simulink model "gm_soc_dvbs2_fpga"  (R2025b)
settings: Solver=VariableStepAuto  StartTime=0.0  StopTime=10.0  RelTol=1e-3
InitFcn:
  | soc_dvbs2_init;
undefined symbols (not defined in the file or in its folder): Add, coefficientsLog, coefficientsSqrt1, coefficientsSqrt2, dataBits, Deinterleaver, designMultirateFIR, noisePow, Shift, Short, soc_dvbs2_designFIRFilter, soc_dvbs2_txPacketBits, syncWord, txDataOut, txFiltCoeff, XData
libraries: simulink x304, hdlsllib x265, dspsigops x15, dsphdlfiltering2 x8, hdlmdlgenlib x6, dsphdlsigops2 x5, commseqgen3 x5, dsphdlmathfun2 x3, hwlogicconnlib x2, whdledac x2, commhdlcrc x2, whdlutilities x1
(part 2 of 36)

== system gm_soc_dvbs2_fpga/DVBS2/DVBS2 TxRx/LUT Based Tx ==
  modcodidx : Inport  OutDataTypeStr=fixdt(0, 5, 0)  PortDimensions=1  SampleTime=2.5e-07
  Constant : Constant  OutDataTypeStr=boolean  SampleTime=2.5e-07
  Data Type Conversion1 : DataTypeConversion  OutDataTypeStr=fixdt(1, 18, 15)  SampleTime=6.25e-08  SaturateOnIntegerOverflow=off  RndMeth=Floor
  Delay : Delay  DelayLength=double(2)  InitialCondition=0  SampleTime=2.5e-07
  Delay1 : Delay  DelayLength=double(1)  InitialCondition=0  SampleTime=2.5e-07
  Delay_out1_wire : RateTransition  Integrity=off  Deterministic=off  OutPortSampleTimeOpt=Multiple of input port sample time  OutPortSampleTimeMultiple=1/4
  Discrete FIR Filter HDL Optimized : dsphdlfiltering2/Discrete FIR Filter  NumeratorSource=Property  Numerator=txFiltCoeff  NumeratorPrototype=[]  FilterStructure=Direct form systolic  SerializationOption=Minimum number of cycles between valid input samples  NumCycles=2  NumberOfMultipliers=2  SimulateUsing=Code generation  roundingMode=Floor  overflowMode=off  CoefficientsDataTypeStr=Inherit: Same word length as input  OutputDataTypeStr=Inherit: Same word length as input  ResetInputPort=off  HDLGlobalReset=off  CoeffMultiplier=Multiplier  UseMultForPow2Coeff=on  FrameInputSymmOptim=off
  Subsystem1 : Subsystem
  Upsample : dspsigops/Upsample  FactorSource=Dialog parameter  N=double(4)  Nmax=16  phase=double(0)  RateOptions=Allow multirate processing  ic=0  mode=Unused parameter value
  txDataOut : Outport  SampleTime=6.25e-08
  txValidOut : Outport  Port=2  SampleTime=6.25e-08
  wires:
  Subsystem1/1(Out1) -> Delay1/1
  modcodidx/1 -> Subsystem1/1(modcodidx)
  Constant/1 -> Delay/1, Subsystem1/2(enb)
  Delay1/1 -> Upsample/1
  Delay_out1_wire/1 -> Discrete FIR Filter HDL Optimized/2
  Delay/1 -> Delay_out1_wire/1
  Discrete FIR Filter HDL Optimized/1 -> Data Type Conversion1/1
  Upsample/1 -> Discrete FIR Filter HDL Optimized/1
  Discrete FIR Filter HDL Optimized/2 -> txValidOut/1
  Data Type Conversion1/1 -> txDataOut/1

== system gm_soc_dvbs2_fpga/DVBS2/DVBS2 TxRx/Prepare Inputs ==
  rxData : Inport  OutDataTypeStr=int16  PortDimensions=1  SampleTime=7.8125e-09
      settings: SignalType=complex
  rxValid : Inport  Port=2  OutDataTypeStr=boolean  PortDimensions=1  SampleTime=7.8125e-09
  Data Type Conversion : DataTypeConversion  OutDataTypeStr=fixdt(1,16,14)  ConvertRealWorld=Stored Integer (SI)  SaturateOnIntegerOverflow=off  RndMeth=Floor
  Data Type Conversion1 : DataTypeConversion  OutDataTypeStr=fixdt(1,18,15)  ConvertRealWorld=Stored Integer (SI)  SaturateOnIntegerOverflow=off  RndMeth=Floor
  Delay{,1..3} (4 alike) : Delay
  Discrete FIR Filter HDL Optimized1 : dsphdlfiltering2/Discrete FIR Filter  NumeratorSource=Property  Numerator=soc_dvbs2_designFIRFilter(32,1.35,8-1.35)  NumeratorPrototype=[]  FilterStructure=Direct form systolic  SerializationOption=Minimum number of cycles between valid input samples  NumCycles=2  NumberOfMultipliers=2  SimulateUsing=Code generation  roundingMode=Floor  overflowMode=off  CoefficientsDataTypeStr=Inherit: Same word length as input  OutputDataTypeStr=Inherit: Same word length as input  ResetInputPort=off  HDLGlobalReset=off  CoeffMultiplier=Multiplier  UseMultForPow2Coeff=on  FrameInputSymmOptim=off
  Downsample1 : DownSample  N=8  RateOptions=Allow multirate processing
  Downsample2 : DownSample  N=8  RateOptions=Allow multirate processing
  Gain : Gain  Gain=2  ParamDataTypeStr=fixdt(0,3,0)  OutDataTypeStr=fixdt(1, 16, 13)
  rxDataOut : Outport  SampleTime=6.25e-08
  rxValidOut : Outport  Port=2  SampleTime=6.25e-08
  wires:
  rxData/1 -> Data Type Conversion/1
  Delay/1 -> Gain/1
  Downsample1/1 -> Delay1/1
  Delay2/1 -> Data Type Conversion1/1
  Discrete FIR Filter HDL Optimized1/1 -> Downsample2/1
  Gain/1 -> Delay2/1
  rxValid/1 -> Discrete FIR Filter HDL Optimized1/2
  Data Type Conversion/1 -> Discrete FIR Filter HDL Optimized1/1
  Downsample2/1 -> Delay/1
  Discrete FIR Filter HDL Optimized1/2 -> Downsample1/1
  Delay1/1 -> Delay3/1
  Delay3/1 -> rxValidOut/1
  Data Type Conversion1/1 -> rxDataOut/1

== system gm_soc_dvbs2_fpga/DVBS2/DVBS2 TxRx/Prepare Outputs ==
  note: Gain
  txData : Inport  OutDataTypeStr=fixdt(1, 18, 15)  PortDimensions=1  SampleTime=6.25e-08
      settings: SignalType=complex
  txvalid : Inport  Port=2  OutDataTypeStr=boolean  PortDimensions=1  SampleTime=6.25e-08
  Data Type Conversion2 : DataTypeConversion  OutDataTypeStr=int16  ConvertRealWorld=Stored Integer (SI)  SaturateOnIntegerOverflow=off  RndMeth=Floor
  Data Type Conversion3 : DataTypeConversion  OutDataTypeStr=fixdt(1,16,13)  SaturateOnIntegerOverflow=off  RndMeth=Floor
  Delay{4..7} (4 alike) : Delay
  Discrete FIR Filter HDL Optimized : dsphdlfiltering2/Discrete FIR Filter  NumeratorSource=Property  Numerator=soc_dvbs2_designFIRFilter(32,1.35,8-1.35)  NumeratorPrototype=[]  FilterStructure=Direct form systolic  SerializationOption=Minimum number of cycles between valid input samples  NumCycles=2  NumberOfMultipliers=2  SimulateUsing=Code generation  roundingMode=Floor  overflowMode=off  CoefficientsDataTypeStr=Inherit: Same word length as input  OutputDataTypeStr=Inherit: Same word length as input  ResetInputPort=off  HDLGlobalReset=off  CoeffMultiplier=Multiplier  UseMultForPow2Coeff=on  FrameInputSymmOptim=off
  Gain : Gain  Gain=8  ParamDataTypeStr=fixdt(0,4,0)  OutDataTypeStr=fixdt(1, 18, 14)
  Repeat : dspsigops/Repeat  FactorSource=Dialog parameter  N=8  Nmax=16  RateOptions=Allow multirate processing  ic=0  mode=Unused parameter value
  Upsample : dspsigops/Upsample  FactorSource=Dialog parameter  N=8  Nmax=16  phase=0  RateOptions=Allow multirate processing  ic=0  mode=Unused parameter value
  txDataOut : Outport  SampleTime=7.8125e-09
  txValidOut : Outport  Port=2  SampleTime=7.8125e-09
  wires:
  txData/1 -> Upsample/1
  txvalid/1 -> Repeat/1
  Delay6/1 -> Delay7/1
  Delay4/1 -> Gain/1
  Discrete FIR Filter HDL Optimized/2 -> Delay6/1
  Upsample/1 -> Discrete FIR Filter HDL Optimized/1
  Discrete FIR Filter HDL Optimized/1 -> Delay4/1
  Repeat/1 -> Discrete FIR Filter HDL Optimized/2
  Gain/1 -> Delay5/1
  Delay7/1 -> txValidOut/1
  Delay5/1 -> Data Type Conversion3/1
  Data Type Conversion3/1 -> Data Type Conversion2/1
  Data Type Conversion2/1 -> txDataOut/1

== system gm_soc_dvbs2_fpga/DVBS2/Vector Decimation/Vector Decimation ==
  din_real : Inport  OutDataTypeStr=int16  PortDimensions=[4]  SampleTime=7.8125e-09
  din_img : Inport  Port=2  OutDataTypeStr=int16  PortDimensions=[4]  SampleTime=7.8125e-09
  vin : Inport  Port=3  OutDataTypeStr=boolean  PortDimensions=1  SampleTime=7.8125e-09
  FIR Decimation HDL Optimized : dsphdlfiltering2/FIR Decimator  NumeratorSource=Property  Numerator=designMultirateFIR(1,4)  NumeratorPrototype=[]  FilterStructure=Direct form systolic  DecimationFactor=4  NumCycles=1  OptimizeSymmCoeff=off  SimulateUsing=Code generation  roundingMode=Floor  overflowMode=off  CoefficientsDataTypeStr=Inherit: Same word length as input  OutputDataTypeStr=fixdt(1,16,0)  ResetInputPort=off  HDLGlobalReset=off
  Real-Imag to Complex : RealImagToComplex
  dout : Outport  SampleTime=7.8125e-09  VectorParamsAs1DForOutWhenUnconnected=off
  vout : Outport  Port=2  SampleTime=7.8125e-09  VectorParamsAs1DForOutWhenUnconnected=off
  wires:
  FIR Decimation HDL Optimized/2 -> vout/1
  vin/1 -> FIR Decimation HDL Optimized/2
  din_real/1 -> Real-Imag to Complex/1
  FIR Decimation HDL Optimized/1 -> dout/1
  din_img/1 -> Real-Imag to Complex/2
  Real-Imag to Complex/1 -> FIR Decimation HDL Optimized/1

== system gm_soc_dvbs2_fpga/DVBS2/BER/Send Payload Data/1-D Lookup Table ==
  In1 : Inport
  1-D Lookup Table : Lookup_n-D  NumberOfTableDimensions=1  LookupTableObject=''  BreakpointsSpecification=Even spacing  BreakpointsForDimension1=0:length(dataBits)-1  BreakpointsForDimension1FirstPoint=0  BreakpointsForDimension2FirstPoint=10  BreakpointsForDimension2Spacing=12  IndexSearchMethod=Evenly spaced points  Table=[syncWord;soc_dvbs2_txPacketBits]  TableDataTypeStr=int8  InterpMethod=Flat  InternalRulePriority=Speed  OutDataTypeStr=int8  RndMeth=Simplest
  1-D Lookup Table_pd1 : Delay  DelayLength=1
  Out1 : Outport
  wires:
  1-D Lookup Table/1 -> 1-D Lookup Table_pd1/1
  In1/1 -> 1-D Lookup Table/1
  1-D Lookup Table_pd1/1 -> Out1/1

== system gm_soc_dvbs2_fpga/DVBS2/DVBS2 TxRx/Channel/AWGN Generator ==
  snrdB : Inport  OutDataTypeStr=fixdt(1, 16, 9)  PortDimensions=1  SampleTime=6.25e-08
  Delay1 : Delay  DelayLength=46
  Gaussian Noise With Given Variance : Subsystem
  Unit Variance Gaussian Noise : Subsystem
  dB to Linear Scale Converter : Subsystem
  awgn : Outport  SampleTime=6.25e-08
  wires:
  snrdB/1 -> dB to Linear Scale Converter/1(snrdB)
  dB to Linear Scale Converter/1(noiseVar) -> Delay1/1
  Gaussian Noise With Given Variance/1(awgn) -> awgn/1
  Unit Variance Gaussian Noise/1(x0) -> Gaussian Noise With Given Variance/2(x0)
  Delay1/1 -> Gaussian Noise With Given Variance/1(noiseVar)
  Unit Variance Gaussian Noise/2(x1) -> Gaussian Noise With Given Variance/3(x1)

== system gm_soc_dvbs2_fpga/DVBS2/DVBS2 TxRx/DVB-S2 HDL Receiver/Demod Deinterleave and FECDecode ==
  dataIn : Inport  OutDataTypeStr=fixdt(1, 18, 14)  PortDimensions=1  SampleTime=7.8125e-09
      settings: SignalType=complex
  validIn : Inport  Port=2  OutDataTypeStr=boolean  PortDimensions=1  SampleTime=7.8125e-09
  endOfPLSC : Inport  Port=3  OutDataTypeStr=boolean  PortDimensions=1  SampleTime=7.8125e-09
  MODCOD : Inport  Port=4  OutDataTypeStr=fixdt(0, 5, 0)  PortDimensions=1  SampleTime=7.8125e-09
  DVBS2 HDL Deinterleaver : Subsystem  mask{mode=Deinterleaver, Tsamp=double(-1)}
      mask prompts: mode "Mode :"; Tsamp "Sample Time"
      mask init:
      | ConfigRx = struct('RAMCapacity', double(129600), 'ShortFrameLen', double(16200), 'NormalFrameLen', double(64800));
      | Tsamp = double(-1);
      | isInterleave = double(0);
      mask TypeOptions mode: Interleaver | Deinterleaver
      mask Display: disp(['DVB-S2' newline 'HDL ' newline get_param(gcb,'mode')]);
  Data Type Conversion3 : DataTypeConversion  OutDataTypeStr=fixdt(1,8,4)  RndMeth=Floor
  Discard Unsupported Frames : Subsystem
  FEC Decoding : Subsystem
  Symbol Demodulaor : Subsystem
  bitsOut : Outport  SampleTime=7.8125e-09
  ctrl : Outport  Port=2
  wires:
  MODCOD/1 -> Discard Unsupported Frames/4(MODCOD)
  validIn/1 -> Discard Unsupported Frames/3(validIn)
  dataIn/1 -> Discard Unsupported Frames/2(dataIn)
  endOfPLSC/1 -> Discard Unsupported Frames/1(endOfPLSC)
  Data Type Conversion3/1 -> DVBS2 HDL Deinterleaver/1(dataIn)
  Discard Unsupported Frames/4(modIdx) -> Symbol Demodulaor/4(modIdx)
  Discard Unsupported Frames/3(paramCapture) -> Symbol Demodulaor/3(paramCapture)
  Discard Unsupported Frames/2(validOut) -> Symbol Demodulaor/2(validIn)
  Discard Unsupported Frames/1(dataOut) -> Symbol Demodulaor/1(dataIn)
  Discard Unsupported Frames/5(codIdx) -> Symbol Demodulaor/5(codIdx)
  Discard Unsupported Frames/6(FECFrameOut) -> Symbol Demodulaor/6(FECFrame)
  Symbol Demodulaor/1(softBitsOut) -> Data Type Conversion3/1
  Symbol Demodulaor/2(validOut) -> DVBS2 HDL Deinterleaver/2(validIn)
  Symbol Demodulaor/3(paramCaptureOut) -> DVBS2 HDL Deinterleaver/3(paramValid)
  Symbol Demodulaor/4(modIdxOut) -> DVBS2 HDL Deinterleaver/4(modIdxIn)
  Symbol Demodulaor/5(codIdxOut) -> DVBS2 HDL Deinterleaver/5(codIdxIn)
  Symbol Demodulaor/6(fecframeOut) -> DVBS2 HDL Deinterleaver/6(fecframeIn)
  DVBS2 HDL Deinterleaver/1(rd_dout) -> FEC Decoding/1(dataIn)
  DVBS2 HDL Deinterleaver/2(rd_startOut) -> FEC Decoding/2(startIn)
  DVBS2 HDL Deinterleaver/3(rd_endOut) -> FEC Decoding/3(endIn)
  DVBS2 HDL Deinterleaver/4(rd_validOut) -> FEC Decoding/4(validIn)
  DVBS2 HDL Deinterleaver/5(fecframe) -> FEC Decoding/5(FECFrame)
  FEC Decoding/2(ctrl) -> ctrl/1
  DVBS2 HDL Deinterleaver/6(codIdx) -> FEC Decoding/6(codIdx)
  FEC Decoding/1(bitsOut) -> bitsOut/1

== system gm_soc_dvbs2_fpga/DVBS2/DVBS2 TxRx/DVB-S2 HDL Receiver/Stream Recovery ==
  bitsIn : Inport  OutDataTypeStr=boolean  PortDimensions=1  SampleTime=7.8125e-09
  startIn : Inport  Port=2  OutDataTypeStr=boolean  PortDimensions=1  SampleTime=7.8125e-09
  validIn : Inport  Port=3  OutDataTypeStr=boolean  PortDimensions=1  SampleTime=7.8125e-09
  BB Decoder : Subsystem
  BB Demultiplexer : Subsystem
  BB Descrambler : Subsystem
  BB Header CRC Check : Subsystem
  Delay{1..2,4..9,11..15,17..18,20..24} (20 alike) : Delay  DelayLength=1
  bitsOut : Outport  OutDataTypeStr=boolean  PortDimensions=[1 1]  SampleTime=7.8125e-09
  startOut : Outport  Port=2  OutDataTypeStr=boolean  PortDimensions=[1 1]  SampleTime=7.8125e-09
  endOut : Outport  Port=3  OutDataTypeStr=boolean  PortDimensions=[1 1]  SampleTime=7.8125e-09
  validOut : Outport  Port=4  OutDataTypeStr=boolean  PortDimensions=[1 1]  SampleTime=7.8125e-09
  invalidPkt : Outport  Port=5  OutDataTypeStr=boolean  PortDimensions=[1 1]  SampleTime=7.8125e-09
  TSorGS : Outport  Port=6  OutDataTypeStr=fixdt(0,2,0)  PortDimensions=[1 1]  SampleTime=7.8125e-09
  SISorMIS : Outport  Port=7  OutDataTypeStr=boolean  PortDimensions=[1 1]  SampleTime=7.8125e-09
  CCMorACM : Outport  Port=8  OutDataTypeStr=boolean  PortDimensions=[1 1]  SampleTime=7.8125e-09
  ISSYI : Outport  Port=9  OutDataTypeStr=boolean  PortDimensions=[1 1]  SampleTime=7.8125e-09
  NPD : Outport  Port=10  OutDataTypeStr=boolean  PortDimensions=[1 1]  SampleTime=7.8125e-09
  RO : Outport  Port=11  OutDataTypeStr=fixdt(0,2,0)  PortDimensions=[1 1]  SampleTime=7.8125e-09
  MIS_ISI : Outport  Port=12  OutDataTypeStr=uint8  PortDimensions=1  SampleTime=7.8125e-09
  UPL : Outport  Port=13  OutDataTypeStr=uint16  PortDimensions=1  SampleTime=7.8125e-09
  DFL : Outport  Port=14  OutDataTypeStr=uint16  PortDimensions=1  SampleTime=7.8125e-09
  SYNC : Outport  Port=15  OutDataTypeStr=uint8  PortDimensions=1  SampleTime=7.8125e-09
  SYNCD : Outport  Port=16  OutDataTypeStr=uint16  PortDimensions=1  SampleTime=7.8125e-09
  wires:
  Delay6/1 -> BB Descrambler/3(validIn)
  BB Header CRC Check/1(dstartOut) -> Delay9/1
  bitsIn/1 -> Delay1/1
  startIn/1 -> Delay2/1
  validIn/1 -> Delay6/1
  Delay17/1 -> BB Demultiplexer/3(validIn)
  BB Descrambler/1(bitsOut) -> Delay7/1
  Delay1/1 -> BB Descrambler/1(bitsIn)
  Delay2/1 -> BB Descrambler/2(startIn)
  Delay15/1 -> BB Demultiplexer/2(startIn)
  BB Descrambler/2(startOut) -> Delay15/1
  BB Descrambler/3(validOut) -> Delay17/1
  Delay7/1 -> BB Demultiplexer/1(bitsIn)
  BB Decoder/5(TSorGS) -> TSorGS/1
  BB Demultiplexer/1(dstartOut) -> Delay18/1
  BB Decoder/12(UPL) -> UPL/1
  BB Demultiplexer/2(dValidOut) -> Delay20/1
  BB Decoder/15(SYNCD) -> SYNCD/1
  BB Demultiplexer/3(bitsOut) -> Delay21/1
  BB Decoder/6(SISorMIS) -> SISorMIS/1
  BB Demultiplexer/4(hstartOut) -> Delay22/1
  BB Decoder/9(NPD) -> NPD/1
  BB Demultiplexer/5(hendOut) -> Delay23/1
  BB Decoder/8(ISSYI) -> ISSYI/1
  BB Demultiplexer/6(hvalidOut) -> Delay24/1
  Delay18/1 -> BB Header CRC Check/1(dstartIn)
  Delay11/1 -> BB Decoder/2(dvalidIn)
  Delay20/1 -> BB Header CRC Check/2(dValidIn)
  Delay21/1 -> BB Header CRC Check/3(bitsIn)
  Delay9/1 -> BB Decoder/1(dstartIn)
  Delay22/1 -> BB Header CRC Check/4(hstartIn)
  Delay23/1 -> BB Header CRC Check/5(hendIn)
  Delay24/1 -> BB Header CRC Check/6(hvalidIn)
  BB Header CRC Check/2(dvalidIn) -> Delay11/1
  BB Header CRC Check/3(dbitsOut) -> Delay8/1
  BB Header CRC Check/4(hbitsOut) -> Delay13/1
  BB Header CRC Check/5(hstartOut) -> Delay4/1
  BB Header CRC Check/6(hendOut) -> Delay5/1
  BB Header CRC Check/7(hvalidOut) -> Delay12/1
  Delay5/1 -> BB Decoder/6(hendIn)
  BB Header CRC Check/8(herrorOut) -> Delay14/1
  Delay8/1 -> BB Decoder/3(dbitsIn)
  Delay13/1 -> BB Decoder/4(hbitsIn)
  Delay4/1 -> BB Decoder/5(hstartIn)
  Delay12/1 -> BB Decoder/7(validIn)
  Delay14/1 -> BB Decoder/8(herrorIn)
  BB Decoder/1(bitsOut) -> bitsOut/1
  BB Decoder/2(startOut) -> startOut/1
  BB Decoder/3(endOut) -> endOut/1
  BB Decoder/4(validOut) -> validOut/1
  BB Decoder/7(CCMorACM) -> CCMorACM/1
  BB Decoder/10(RO) -> RO/1
  BB Decoder/11(MIS_ISI) -> MIS_ISI/1
  BB Decoder/13(DFL) -> DFL/1
  BB Decoder/14(SYNC) -> SYNC/1
  BB Decoder/16(invalidPkt) -> invalidPkt/1

== system gm_soc_dvbs2_fpga/DVBS2/DVBS2 TxRx/DVB-S2 HDL Receiver/Synchronizer and PL Header Decoder ==
  dataIn : Inport  OutDataTypeStr=fixdt(1, 18, 15)  PortDimensions=1  SampleTime=6.25e-08
      settings: SignalType=complex
  validIn : Inport  Port=2  OutDataTypeStr=boolean  PortDimensions=1  SampleTime=6.25e-08
  rstFCPO : Inport  Port=3  OutDataTypeStr=boolean  PortDimensions=1  SampleTime=6.25e-08
  Bus Creator : BusCreator  Inputs=2
  Bus Creator1 : BusCreator  Inputs=2
  Bus Creator2 : BusCreator  Inputs=5
  Delay10 : Delay  DelayLength=6
  Delay{3,11,13..21,24} (12 alike) : Delay  DelayLength=1
  Delay{4..7,12} (5 alike) : Delay
  Delay9 : Delay  DelayLength=6
  Downsample : DownSample  N=config.SamplesPerSymbol  RateOptions=Allow multirate processing
  "Enable MODCOD " : Subsystem
  Fine Phase Synchronizer : Subsystem
  PL Header Recovery : Subsystem
  Source Encoding : Subsystem
  Time Frequency and Coarse Phase Synchronizer : Subsystem
  dataOut : Outport  SampleTime=2.5e-07
  validOut : Outport  Port=2  SampleTime=2.5e-07
  endOfPLSC : Outport  Port=3  SampleTime=2.5e-07
  headerInfo : Outport  Port=4
  diagBus : Outport  Port=5
  wires:
  [diagBus3] -> Bus Creator2/3  "SymbolSyncedSymbols"
  dataIn/1 -> Delay20/1
  Delay7/1 -> Delay10/1
  [diagBus1] -> Bus Creator2/1  "PLSCSymbols"
  [diagBus5] -> Bus Creator2/5  "VisualizeCorrelationSignals"
  Downsample/1 -> Fine Phase Synchronizer/6(rst)
  [diagBus4] -> Bus Creator2/4  "pilotsConstellation"
  [diagBus2] -> Bus Creator2/2  "NormalizedFrequencyEstimates"
  Bus Creator2/1 -> Delay11/1
  PL Header Recovery/4(endOfPLSC) -> Delay5/1
  Time Frequency and Coarse Phase Synchronizer/3(validOut) -> Delay14/1
  validIn/1 -> Delay3/1
  Delay20/1 -> Time Frequency and Coarse Phase Synchronizer/1(dataIn)
  Delay3/1 -> Time Frequency and Coarse Phase Synchronizer/2(validIn)
  Source Encoding/1(mod) -> Fine Phase Synchronizer/4(mod)
  Delay15/1 -> PL Header Recovery/3(endOfSOF)
  Delay11/1 -> diagBus/1
  Delay4/1 -> Fine Phase Synchronizer/2(validIn)
  PL Header Recovery/2(dataOut) -> Delay12/1
  Time Frequency and Coarse Phase Synchronizer/1(finePhaseEn) -> Fine Phase Synchronizer/5(En)
  Time Frequency and Coarse Phase Synchronizer/2(dataOut) -> Delay13/1
  Time Frequency and Coarse Phase Synchronizer/4(endOfSOF) -> Delay15/1
  Time Frequency and Coarse Phase Synchronizer/5(hasPilots) -> Delay16/1
  Time Frequency and Coarse Phase Synchronizer/6(normCoarFreqEst) -> Bus Creator/1  "NormalizedCoarseFrequencyEstimate"
  Time Frequency and Coarse Phase Synchronizer/7(normFineFreqEst) -> Bus Creator/2  "NormalizedFineFrequencyEstimate"
  Time Frequency and Coarse Phase Synchronizer/8(synbSyncDiag) -> [diagBus3]
  Time Frequency and Coarse Phase Synchronizer/9(pilotConstel) -> [diagBus4]
  Time Frequency and Coarse Phase Synchronizer/10(VisualizeCorrelationSignals) -> [diagBus5]
  Time Frequency and Coarse Phase Synchronizer/11(enbMODCOD) -> "Enable MODCOD "/2(enb)
  Delay13/1 -> PL Header Recovery/1(dataIn)
  Delay14/1 -> PL Header Recovery/2(validIn)
  Delay16/1 -> PL Header Recovery/4(hasPilots)
  PL Header Recovery/5(modcod) -> Source Encoding/1(modcod), Delay6/1
  Bus Creator/1 -> [diagBus2]
  Bus Creator1/1 -> Delay21/1
  Delay5/1 -> Fine Phase Synchronizer/3(endOfPLSCIn)
  PL Header Recovery/1(PLSCDiag) -> [diagBus1]
  rstFCPO/1 -> Delay24/1
  PL Header Recovery/3(validOut) -> Delay4/1
  Delay9/1 -> "Enable MODCOD "/1(modcod)
  PL Header Recovery/6(FEC) -> Delay7/1
  Delay24/1 -> Downsample/1
  Delay12/1 -> Fine Phase Synchronizer/1(dataIn)
  Delay6/1 -> Delay9/1
  Fine Phase Synchronizer/1(dataOut) -> Delay17/1
  Fine Phase Synchronizer/2(validOut) -> Delay18/1
  Fine Phase Synchronizer/3(endOfPLSC) -> Delay19/1
  Delay10/1 -> Bus Creator1/2  "FECFrame"
  Delay17/1 -> dataOut/1
  Delay18/1 -> validOut/1
  Delay19/1 -> endOfPLSC/1
  "Enable MODCOD "/1(modcodOut) -> Bus Creator1/1  "MODCOD"
  Delay21/1 -> headerInfo/1

== system gm_soc_dvbs2_fpga/DVBS2/DVBS2 TxRx/Digital Automatic Gain Control/Error Detector ==
  dataIn : Inport  OutDataTypeStr=fixdt(1, 18, 15)  PortDimensions=1  SampleTime=6.25e-08
      settings: SignalType=complex
  Add1 : Sum  Inputs=+-  OutDataTypeStr=fixdt(1, 37, 30)
  Complex to Real-Imag : ComplexToRealImag  Output=Real
  Conj : Math  Operator=conj  OutDataTypeStr=fixdt(1, 18, 15)
  Delay{,1,3..4} (4 alike) : Delay
  Product : Product  OutDataTypeStr=fixdt(1, 36, 30)
  Reference : Constant  Value=desiredOutputPower  OutDataTypeStr=fixdt(1, 18, 15)  SampleTime=-1
  err : Outport  SampleTime=6.25e-08
  wires:
  dataIn/1 -> Delay1/1, Conj/1
  Reference/1 -> Add1/1
  Conj/1 -> Delay/1
  Delay4/1 -> Complex to Real-Imag/1
  Product/1 -> Delay4/1
  Add1/1 -> Delay3/1
  Delay1/1 -> Product/1
  Delay3/1 -> err/1
  Complex to Real-Imag/1 -> Add1/2
  Delay/1 -> Product/2

== system gm_soc_dvbs2_fpga/DVBS2/DVBS2 TxRx/Digital Automatic Gain Control/Loop Filter ==
  err : Inport  OutDataTypeStr=fixdt(1, 37, 30)  PortDimensions=1  SampleTime=6.25e-08
  Add : Sum  OutDataTypeStr=fixdt(1, 37, 30)  AccumDataTypeStr=fixdt(1, 38, 30)  SampleTime=6.25e-08
  Delay1 : Delay  DelayLength=double(1)  InitialCondition=0  SampleTime=6.25e-08
  Delay2 : Delay  DelayLength=double(2)  InitialCondition=0  SampleTime=6.25e-08
  Delay3 : Delay  DelayLength=double(2)  InitialCondition=0  SampleTime=6.25e-08
  Gain1 : Gain  Gain="fi(0,1,37,46,\"hex\",\"083126e979\")"  ParamDataTypeStr=fixdt(1, 37, 46)  OutDataTypeStr=fixdt(1, 37, 30)  SampleTime=6.25e-08
  gain : Outport  SampleTime=6.25e-08
  wires:
  err/1 -> Delay3/1
  Delay1/1 -> gain/1, Add/2
  Delay3/1 -> Gain1/1
  Add/1 -> Delay1/1
  Gain1/1 -> Delay2/1
  Delay2/1 -> Add/1

== system gm_soc_dvbs2_fpga/DVBS2/DVBS2 TxRx/LUT Based Tx/Subsystem1 ==
  modcodidx : Inport  OutDataTypeStr=fixdt(0, 5, 0)  PortDimensions=1  SampleTime=2.5e-07
  enb : Inport  Port=2  OutDataTypeStr=boolean  PortDimensions=1  SampleTime=2.5e-07
  Delay : Delay  DelayLength=double(1)  InitialCondition=0  SampleTime=2.5e-07
  From : hdlmdlgenlib/Buffer
  Goto : hdlmdlgenlib/Buffer
  Logical Operator : Logic  Operator=OR  Inputs=4  AllPortsSameDT=off  OutDataTypeStr=boolean  SampleTime=2.5e-07
  Multiport Switch : MultiPortSwitch  DataPortOrder=Zero-based contiguous  Inputs=24  DataPortForDefault=Additional data port  DiagnosticForDefault=None  zeroidx=on  OutDataTypeStr=fixdt(1, 18, 16)  SampleTime=2.5e-07  SaturateOnIntegerOverflow=off  InputSameDT=off
  Subsystem : Subsystem
  Subsystem1 : Subsystem
  Subsystem2 : Subsystem
  Subsystem4 : Subsystem
  Unit Delay Enabled Synchronous : hdlsllib/Discrete/Unit Delay Enabled Synchronous  InitialCondition=double(0)  SampleTime=-1
  delayMatch : Delay  DelayLength=double(1)  InitialCondition=0  SampleTime=2.5e-07
  Out1 : Outport  SampleTime=2.5e-07
  wires:
  Subsystem/2(Out3) -> Multiport Switch/3
  Subsystem/6(Out7) -> Multiport Switch/7
  modcodidx/1 -> Unit Delay Enabled Synchronous/1
  From/1 -> Subsystem1/3(modcodidx), Subsystem/3(modcodidx), Subsystem4/3(modcodidx), Subsystem2/3(modcodidx)
  Subsystem4/7(Out1) -> Logical Operator/2
  Goto/1 -> From/1
  Unit Delay Enabled Synchronous/1 -> delayMatch/1, Goto/1
  delayMatch/1 -> Multiport Switch/1
  Subsystem/1(Out2) -> Multiport Switch/26, Multiport Switch/2
  Subsystem/5(Out6) -> Multiport Switch/6
  enb/1 -> Subsystem2/2(enb), Subsystem4/2(enb), Subsystem1/2(enb), Subsystem/2(enb)
  Subsystem/3(Out4) -> Multiport Switch/4
  Subsystem/4(Out5) -> Multiport Switch/5
  Subsystem/7(Out1) -> Logical Operator/1
  Subsystem1/1(Out2) -> Multiport Switch/8
  Subsystem1/2(Out3) -> Multiport Switch/9
  Subsystem1/3(Out4) -> Multiport Switch/10
  Subsystem1/4(Out5) -> Multiport Switch/11
  Subsystem1/5(Out6) -> Multiport Switch/12
  Subsystem1/6(Out7) -> Multiport Switch/13
  Subsystem1/7(Out1) -> Logical Operator/3
  Subsystem4/1(Out2) -> Multiport Switch/14
  Subsystem4/2(Out3) -> Multiport Switch/15
  Subsystem4/3(Out4) -> Multiport Switch/16
  Subsystem4/4(Out5) -> Multiport Switch/17
  Subsystem4/5(Out6) -> Multiport Switch/18
  Subsystem4/6(Out7) -> Multiport Switch/19
  Subsystem2/1(Out2) -> Multiport Switch/20
  Delay/1 -> Subsystem2/1(rst), Subsystem4/1(rst), Subsystem/1(rst), Subsystem1/1(rst)
  Subsystem2/2(Out3) -> Multiport Switch/21
  Subsystem2/3(Out4) -> Multiport Switch/22
  Subsystem2/4(Out5) -> Multiport Switch/23
  Subsystem2/5(Out6) -> Multiport Switch/24
  Subsystem2/6(Out7) -> Multiport Switch/25
  Subsystem2/7(Out1) -> Logical Operator/4
  Multiport Switch/1 -> Out1/1
  Logical Operator/1 -> Unit Delay Enabled Synchronous/2, Delay/1

== system gm_soc_dvbs2_fpga/DVBS2/DVBS2 TxRx/Channel/AWGN Generator/Gaussian Noise With Given Variance ==
  noiseVar : Inport  OutDataTypeStr=fixdt(0, 22, 18)  PortDimensions=1  SampleTime=6.25e-08
  x0 : Inport  Port=2  OutDataTypeStr=fixdt(1, 16, 11)  PortDimensions=1  SampleTime=6.25e-08
  x1 : Inport  Port=3  OutDataTypeStr=fixdt(1, 16, 11)  PortDimensions=1  SampleTime=6.25e-08
  Add1 : Sum  OutDataTypeStr=fixdt(1, 16, 11)  AccumDataTypeStr=fixdt(1, 33, 25)  SampleTime=6.25e-08
  Delay{1..9} (9 alike) : Delay  DelayLength=double(2)  InitialCondition=0  SampleTime=6.25e-08
  Gain : Gain  Gain="fi(0,1,16,14,\"hex\",\"0000 + 4000 i\")"  ParamDataTypeStr=fixdt(1, 16, 14)  OutDataTypeStr=fixdt(1, 32, 25)  SampleTime=6.25e-08
  Product1 : Product  Inputs=**  OutDataTypeStr=fixdt(1, 38, 29)  SampleTime=6.25e-08
  Product11 : Product  Inputs=**  OutDataTypeStr=fixdt(1, 38, 29)  SampleTime=6.25e-08
  Product1_C2ReIm : ComplexToRealImag  SampleTime=6.25e-08
  Product1_ReIm2Complex : RealImagToComplex  SampleTime=6.25e-08
  awgn : Outport  SampleTime=6.25e-08
  wires:
  Delay5/1 -> Add1/2
  x1/1 -> Delay9/1
  Delay4/1 -> Add1/1
  Delay3/1 -> Product1_C2ReIm/1
  x0/1 -> Delay8/1
  Product11/1 -> Product1_ReIm2Complex/2
  Product1_C2ReIm/2 -> Product11/1
  Gain/1 -> Delay5/1
  Delay8/1 -> Delay4/1
  Delay9/1 -> Gain/1
  noiseVar/1 -> Delay7/1
  Product1_ReIm2Complex/1 -> Delay1/1
  Product1/1 -> Product1_ReIm2Complex/1
  Add1/1 -> Delay3/1
  Delay7/1 -> Delay6/1
  Delay6/1 -> Delay2/1
  Product1_C2ReIm/1 -> Product1/1
  Delay2/1 -> Product11/2, Product1/2
  Delay1/1 -> awgn/1

== system gm_soc_dvbs2_fpga/DVBS2/DVBS2 TxRx/Channel/AWGN Generator/Unit Variance Gaussian Noise ==
  Delay{,1..2,31,33} (5 alike) : Delay  DelayLength=double(1)  InitialCondition=0  SampleTime=6.25e-08
  Delay{5..10} (6 alike) : Delay  DelayLength=double(2)  InitialCondition=0  SampleTime=6.25e-08
  Delay23 : Delay  DelayLength=double(19)  InitialCondition=0  SampleTime=6.25e-08
  Delay24 : Delay  DelayLength=double(19)  InitialCondition=0  SampleTime=6.25e-08
  Delay3 : Delay  DelayLength=double(21)  InitialCondition=0  SampleTime=6.25e-08
  Delay4 : Delay  DelayLength=double(21)  InitialCondition=0  SampleTime=6.25e-08
  Product : Product  Inputs=**  OutDataTypeStr=fixdt(1, 33, 28)  SampleTime=6.25e-08
  Product1 : Product  Inputs=**  OutDataTypeStr=fixdt(1, 33, 28)  SampleTime=6.25e-08
  Product1_out_dtc : DataTypeConversion  OutDataTypeStr=fixdt(1, 16, 11)  SampleTime=6.25e-08  SaturateOnIntegerOverflow=off  RndMeth=Floor
  Product_out_dtc : DataTypeConversion  OutDataTypeStr=fixdt(1, 16, 11)  SampleTime=6.25e-08  SaturateOnIntegerOverflow=off  RndMeth=Floor
  SinCos : Subsystem
  SqrtImplementation : Subsystem
  TausUniformRandGen : Subsystem
  logImplementation : Subsystem
  x0 : Outport  SampleTime=6.25e-08
  x1 : Outport  Port=2  SampleTime=6.25e-08
  wires:
  TausUniformRandGen/1(u0(16,16)) -> Delay/1
  Delay1/1 -> SqrtImplementation/1(u)
  Delay/1 -> logImplementation/1(u0(48,48))
  TausUniformRandGen/2(u1(16,16)) -> Delay2/1
  Delay2/1 -> SinCos/1(u1)
  logImplementation/1(e) -> Delay1/1
  SinCos/2(g1(16,15)) -> Delay4/1
  SinCos/1(g0) -> Delay3/1
  Delay9/1 -> x0/1
  SqrtImplementation/1(f) -> Delay7/1, Delay5/1
  Delay3/1 -> Delay31/1
  Delay4/1 -> Delay33/1
  Delay31/1 -> Delay23/1
  Delay33/1 -> Delay24/1
  Delay23/1 -> Delay6/1
  Delay8/1 -> Product1/2
  Delay24/1 -> Delay8/1
  Delay5/1 -> Product/1
  Delay6/1 -> Product/2
  Delay7/1 -> Product1/1
  Product/1 -> Product_out_dtc/1
  Product1/1 -> Product1_out_dtc/1
  Product_out_dtc/1 -> Delay9/1
  Product1_out_dtc/1 -> Delay10/1
  Delay10/1 -> x1/1

== system gm_soc_dvbs2_fpga/DVBS2/DVBS2 TxRx/Channel/AWGN Generator/dB to Linear Scale Converter ==
  snrdB : Inport  OutDataTypeStr=fixdt(1, 16, 9)  PortDimensions=1  SampleTime=6.25e-08
  Add : Sum  OutDataTypeStr=int16  AccumDataTypeStr=int16  SampleTime=6.25e-08
  Constant : Constant  Value=201  OutDataTypeStr=int16  SampleTime=6.25e-08
  Delay{1..4} (4 alike) : Delay  DelayLength=double(2)  InitialCondition=0  SampleTime=6.25e-08
  Delay5 : Delay  DelayLength=double(1)  InitialCondition=0  SampleTime=6.25e-08
  Delay6 : Delay  DelayLength=double(1)  InitialCondition=0  SampleTime=6.25e-08
  Gain : Gain  Gain="fi(0,1,16,11,\"hex\",\"5000\")"  ParamDataTypeStr=fixdt(1, 16, 11)  OutDataTypeStr=fixdt(1, 32, 20)  SampleTime=6.25e-08
  Gain_out_dtc : DataTypeConversion  OutDataTypeStr=int16  RndMeth=Round  SampleTime=6.25e-08  SaturateOnIntegerOverflow=off
  sqrt(noisePow/2) : Lookup_n-D  NumberOfTableDimensions=1  LookupTableObject=''  BreakpointsForDimension1=0:511  BreakpointsForDimension1FirstPoint=10  BreakpointsForDimension2FirstPoint=10  BreakpointsForDimension1Spacing=12  BreakpointsForDimension2Spacing=12  IndexSearchMethod=Evenly spaced points  Table=[0 noisePow]  InterpMethod=Flat  InternalRulePriority=Speed  OutDataTypeStr=fixdt(0,22,18)  RndMeth=Simplest
  noiseVar : Outport  SampleTime=6.25e-08
  wires:
  Constant/1 -> Add/2
  Delay3/1 -> Add/1
  Delay2/1 -> Gain/1
  snrdB/1 -> Delay5/1
  Add/1 -> Delay1/1
  Gain_out_dtc/1 -> Delay3/1
  Gain/1 -> Gain_out_dtc/1
  Delay5/1 -> Delay2/1
  Delay1/1 -> sqrt(noisePow/2)/1
  sqrt(noisePow/2)/1 -> Delay4/1
  Delay4/1 -> Delay6/1
  Delay6/1 -> noiseVar/1

== system gm_soc_dvbs2_fpga/DVBS2/DVBS2 TxRx/DVB-S2 HDL Receiver/Demod Deinterleave and FECDecode/DVBS2 HDL Deinterleaver ==
  dataIn : Inport  OutDataTypeStr=fixdt(1, 8, 4)  PortDimensions=1  SampleTime=7.8125e-09
  validIn : Inport  Port=2  OutDataTypeStr=boolean  PortDimensions=1  SampleTime=7.8125e-09
  paramValid : Inport  Port=3  OutDataTypeStr=boolean  PortDimensions=1  SampleTime=7.8125e-09
  modIdxIn : Inport  Port=4  OutDataTypeStr=fixdt(0, 2, 0)  PortDimensions=1  SampleTime=7.8125e-09
  codIdxIn : Inport  Port=5  OutDataTypeStr=fixdt(0, 4, 0)  PortDimensions=1  SampleTime=7.8125e-09
  fecframeIn : Inport  Port=6  OutDataTypeStr=boolean  PortDimensions=1  SampleTime=7.8125e-09
  Constant1 : Constant  Value=0  OutDataTypeStr=fixdt(1, 8, 4)  SampleTime=Tsamp
  Delay{,1..15,20..23} (20 alike) : Delay  DelayLength=1
  Delay16 : Delay  DelayLength=4
  Delay17 : Delay  DelayLength=4
  Discard Out of  Frame samples : Subsystem
  RAM : Subsystem
  RAM Address Generator : Subsystem
  Switch : Switch  Criteria=u2 > Threshold  OutDataTypeStr=fixdt(1, 8, 4)  SaturateOnIntegerOverflow=off  InputSameDT=off
  Unit Delay Enabled Synchronous : hdlsllib/Discrete/Unit Delay Enabled Synchronous  InitialCondition=0.0  SampleTime=-1
  Unit Delay Enabled Synchronous1 : hdlsllib/Discrete/Unit Delay Enabled Synchronous  InitialCondition=0.0  SampleTime=-1
  Unit Delay Enabled Synchronous2 : hdlsllib/Discrete/Unit Delay Enabled Synchronous  InitialCondition=0.0  SampleTime=-1
  codIdxReg : hdlsllib/Discrete/Unit Delay Enabled Synchronous  InitialCondition=0.0  SampleTime=-1
  fecframeReg : hdlsllib/Discrete/Unit Delay Enabled Synchronous  InitialCondition=0.0  SampleTime=-1
  rd_dout : Outport  SampleTime=7.8125e-09
  rd_startOut : Outport  Port=2  SampleTime=7.8125e-09
  rd_endOut : Outport  Port=3  SampleTime=7.8125e-09
  rd_validOut : Outport  Port=4  SampleTime=7.8125e-09
  fecframe : Outport  Port=5  SampleTime=7.8125e-09
  codIdx : Outport  Port=6  SampleTime=7.8125e-09
  wires:
  codIdxIn/1 -> Unit Delay Enabled Synchronous2/1
  Delay15/1 -> fecframeReg/1
  fecframeIn/1 -> Unit Delay Enabled Synchronous1/1
  validIn/1 -> Discard Out of  Frame samples/2(valid)
  Delay10/1 -> RAM/4(rd_addr)
  dataIn/1 -> Discard Out of  Frame samples/1(dataIn)
  modIdxIn/1 -> Unit Delay Enabled Synchronous/1
  paramValid/1 -> Unit Delay Enabled Synchronous/2, Delay/1, Unit Delay Enabled Synchronous2/2, Unit Delay Enabled Synchronous1/2, Discard Out of  Frame samples/3(reset)
  Delay/1 -> Delay20/1
  Unit Delay Enabled Synchronous1/1 -> Delay21/1, Discard Out of  Frame samples/4(fec)
  Unit Delay Enabled Synchronous/1 -> Delay22/1
  Unit Delay Enabled Synchronous2/1 -> Delay23/1
  Discard Out of  Frame samples/1(dataOut) -> Delay1/1
  Discard Out of  Frame samples/2(validOut) -> Delay2/1
  RAM/3(rd_endOut) -> rd_endOut/1
  RAM Address Generator/4(readAddr) -> Delay10/1
  Delay21/1 -> Delay6/1
  RAM/4(rd_validOut) -> Switch/2, rd_validOut/1
  RAM Address Generator/5(readValid) -> Delay11/1
  Delay20/1 -> Delay3/1
  RAM Address Generator/3(writeEnable) -> Delay9/1
  Delay22/1 -> Delay4/1
  Delay23/1 -> Delay5/1
  Delay1/1 -> RAM Address Generator/1(dataIn)
  RAM/1(rd_dout) -> Switch/1
  RAM Address Generator/6(readEnd) -> Delay12/1
  Delay2/1 -> RAM Address Generator/2(validIn)
  Delay6/1 -> RAM Address Generator/4(fecframeIn)
  Delay3/1 -> RAM Address Generator/3(paramValid)
  Delay4/1 -> RAM Address Generator/5(modIdxIn)
  Delay5/1 -> RAM Address Generator/6(codIdxIn)
  Delay17/1 -> fecframe/1
  RAM/2(rd_startOut) -> rd_startOut/1
  RAM Address Generator/7(readStart) -> Delay13/1
  RAM Address Generator/1(dataOut) -> Delay7/1
  RAM Address Generator/9(fecframe) -> Delay15/1
  RAM Address Generator/2(writeAddr) -> Delay8/1
  Delay16/1 -> codIdx/1
  RAM Address Generator/8(codIdx) -> Delay14/1
  Delay7/1 -> RAM/1(wr_din)
  Delay8/1 -> RAM/2(wr_addr)
  Delay9/1 -> RAM/3(wr_en)
  Delay11/1 -> RAM/5(rd_valid)
  Delay12/1 -> RAM/6(rd_end)
  Switch/1 -> rd_dout/1
  fecframeReg/1 -> Delay17/1
  Delay13/1 -> codIdxReg/2, RAM/7(rd_start), fecframeReg/2
  Delay14/1 -> codIdxReg/1
  Constant1/1 -> Switch/3
  codIdxReg/1 -> Delay16/1

== system gm_soc_dvbs2_fpga/DVBS2/DVBS2 TxRx/DVB-S2 HDL Receiver/Demod Deinterleave and FECDecode/Discard Unsupported Frames ==
  endOfPLSC : Inport  OutDataTypeStr=boolean  PortDimensions=1  SampleTime=7.8125e-09
  dataIn : Inport  Port=2  OutDataTypeStr=fixdt(1, 18, 14)  PortDimensions=1  SampleTime=7.8125e-09
      settings: SignalType=complex
  validIn : Inport  Port=3  OutDataTypeStr=boolean  PortDimensions=1  SampleTime=7.8125e-09
  MODCOD : Inport  Port=4  OutDataTypeStr=fixdt(0, 5, 0)  PortDimensions=1  SampleTime=7.8125e-09
  Compare To Constant : simulink/Logic and Bit Operations/Compare To Constant  relop===  const=0  OutDataTypeStr=boolean
  Compare To Constant1 : simulink/Logic and Bit Operations/Compare To Constant  relop===  const=11  OutDataTypeStr=boolean
  Compare To Constant2 : simulink/Logic and Bit Operations/Compare To Constant  relop===  const=17  OutDataTypeStr=boolean
  Compare To Constant3 : simulink/Logic and Bit Operations/Compare To Constant  relop===  const=23  OutDataTypeStr=boolean
  Compare To Constant4 : simulink/Logic and Bit Operations/Compare To Constant  relop===  const=28  OutDataTypeStr=boolean
  Compare To Constant5 : simulink/Logic and Bit Operations/Compare To Constant  relop=>  const=28  OutDataTypeStr=boolean
  Constant : Constant  Value=complex(0)  OutDataTypeStr=fixdt(1, 18, 14)  SampleTime=-1
  Constant1 : Constant  OutDataTypeStr=boolean  SampleTime=-1
  Data Type Conversion : DataTypeConversion  OutDataTypeStr=fixdt(0,2,0)  SaturateOnIntegerOverflow=off  RndMeth=Floor
  Data Type Conversion1 : DataTypeConversion  OutDataTypeStr=fixdt(0,4,0)  SaturateOnIntegerOverflow=off  RndMeth=Floor
  Delay10 : Delay  DelayLength=8
  Delay{2..9} (8 alike) : Delay  DelayLength=1
  Logical Operator : Logic  Operator=OR  Inputs=4  AllPortsSameDT=off  OutDataTypeStr=boolean
  Logical Operator1 : Logic  AllPortsSameDT=off  OutDataTypeStr=boolean
  Logical Operator2 : Logic  AllPortsSameDT=off  OutDataTypeStr=boolean
  Logical Operator3 : Logic  Operator=OR  AllPortsSameDT=off  OutDataTypeStr=boolean
  Logical Operator4 : Logic  Operator=OR  AllPortsSameDT=off  OutDataTypeStr=boolean
  Logical Operator5 : Logic  AllPortsSameDT=off  OutDataTypeStr=boolean
  Switch : Switch  Criteria=u2 ~= 0  OutDataTypeStr=fixdt(1, 18, 14)  SaturateOnIntegerOverflow=off  InputSameDT=off
  Unit Delay Enabled Resettable Synchronous : hdlsllib/Discrete/Unit Delay Enabled Resettable Synchronous  InitialCondition=0.0  SampleTime=-1
  Unit Delay Enabled Synchronous : hdlsllib/Discrete/Unit Delay Enabled Synchronous  InitialCondition=0.0  SampleTime=-1
  Unit Delay Enabled Synchronous1 : hdlsllib/Discrete/Unit Delay Enabled Synchronous  InitialCondition=0.0  SampleTime=-1
  convertMODCOD : Subsystem
  dataOut : Outport  SampleTime=7.8125e-09
  validOut : Outport  Port=2  SampleTime=7.8125e-09
  paramCapture : Outport  Port=3  SampleTime=7.8125e-09
  modIdx : Outport  Port=4  SampleTime=7.8125e-09
  codIdx : Outport  Port=5  SampleTime=7.8125e-09
  FECFrameOut : Outport  Port=6  SampleTime=7.8125e-09
  wires:
  Compare To Constant3/1 -> Logical Operator/3
  Compare To Constant2/1 -> Logical Operator/2
  Compare To Constant1/1 -> Logical Operator/1
  Compare To Constant/1 -> Logical Operator4/1
  MODCOD/1 -> Unit Delay Enabled Synchronous/1
  endOfPLSC/1 -> Delay10/1
  Delay10/1 -> Unit Delay Enabled Synchronous1/2, Unit Delay Enabled Synchronous/2, Delay7/1
  Constant1/1 -> Unit Delay Enabled Synchronous1/1
  Compare To Constant4/1 -> Logical Operator/4
  Unit Delay Enabled Synchronous/1 -> Compare To Constant3/1, Compare To Constant1/1, Compare To Constant/1, Compare To Constant4/1, Compare To Constant5/1, Delay3/1, Compare To Constant2/1
  Compare To Constant5/1 -> Logical Operator4/2
  Unit Delay Enabled Synchronous1/1 -> Logical Operator1/2, Delay2/1
  Delay2/1 -> FECFrameOut/1
  Delay3/1 -> convertMODCOD/1(modcod)
  Logical Operator/1 -> Logical Operator1/1
  Logical Operator4/1 -> Logical Operator3/1
  Data Type Conversion1/1 -> codIdx/1
  convertMODCOD/1(modIdx) -> Data Type Conversion/1
  Logical Operator2/1 -> Switch/2, validOut/1
  convertMODCOD/2(codIdx) -> Data Type Conversion1/1
  Logical Operator5/1 -> paramCapture/1
  Logical Operator1/1 -> Logical Operator3/2
  validIn/1 -> Delay5/1
  Data Type Conversion/1 -> modIdx/1
  Delay7/1 -> Unit Delay Enabled Resettable Synchronous/2, Unit Delay Enabled Resettable Synchronous/1, Delay9/1
  Logical Operator3/1 -> Unit Delay Enabled Resettable Synchronous/3
  Delay5/1 -> Delay4/1
  dataIn/1 -> Delay6/1
  Switch/1 -> dataOut/1
  Delay9/1 -> Logical Operator5/1
  Unit Delay Enabled Resettable Synchronous/1 -> Logical Operator5/2, Logical Operator2/2
  Delay4/1 -> Logical Operator2/1
  Delay6/1 -> Delay8/1
  Delay8/1 -> Switch/1
  Constant/1 -> Switch/3

== system gm_soc_dvbs2_fpga/DVBS2/DVBS2 TxRx/DVB-S2 HDL Receiver/Demod Deinterleave and FECDecode/FEC Decoding ==
  dataIn : Inport  OutDataTypeStr=fixdt(1, 8, 4)  PortDimensions=1  SampleTime=7.8125e-09
  startIn : Inport  Port=2  OutDataTypeStr=boolean  PortDimensions=1  SampleTime=7.8125e-09
  endIn : Inport  Port=3  OutDataTypeStr=boolean  PortDimensions=1  SampleTime=7.8125e-09
  validIn : Inport  Port=4  OutDataTypeStr=boolean  PortDimensions=1  SampleTime=7.8125e-09
  FECFrame : Inport  Port=5  OutDataTypeStr=boolean  PortDimensions=1  SampleTime=7.8125e-09
  codIdx : Inport  Port=6  OutDataTypeStr=fixdt(0, 4, 0)  PortDimensions=1  SampleTime=7.8125e-09
  DVB-S2 BCH Decoder : whdledac/DVB-S2 BCH Decoder  FECFrameSource=Property  FECFrameType=Short  CodeRateSource=Input port  CodeRateNormal=1/4  CodeRateShort=1/4  NumErrorsOutputPort=off  SimulateUsing=Code generation
  DVB-S2 BCH Decoder_term2 : Terminator
  DVB-S2 LDPC Decoder : whdledac/DVB-S2 LDPC Decoder  FECFrameSource=Input port  FECFrame=Normal  CodeRateSource=Property  CodeRateNormal=1/4  CodeRateShort=1/4  Parallelism=45  Algorithm=Min-sum  SourceScalingFactor=Property  ScalingFactor=0.75  Termination=Max  SpecifyInputs=Property  NumIterations=8  MaxNumIterations=8  ParityCheckStatus=off  SimulateUsing=Code generation
  DVB-S2 LDPC Decoder_term2 : Terminator
  Sample Control Bus Creator : whdlutilities/Sample Control Bus Creator
  bitsOut : Outport  SampleTime=7.8125e-09
  ctrl : Outport  Port=2
  wires:
  codIdx/1 -> DVB-S2 BCH Decoder/3, DVB-S2 LDPC Decoder/4
  DVB-S2 BCH Decoder/1 -> bitsOut/1
  validIn/1 -> Sample Control Bus Creator/3
  DVB-S2 BCH Decoder/3 -> DVB-S2 BCH Decoder_term2/1
  startIn/1 -> Sample Control Bus Creator/1
  FECFrame/1 -> DVB-S2 LDPC Decoder/3
  Sample Control Bus Creator/1 -> DVB-S2 LDPC Decoder/2
  dataIn/1 -> DVB-S2 LDPC Decoder/1
  endIn/1 -> Sample Control Bus Creator/2
  DVB-S2 LDPC Decoder/1 -> DVB-S2 BCH Decoder/1
  DVB-S2 LDPC Decoder/2 -> DVB-S2 BCH Decoder/2
  DVB-S2 LDPC Decoder/3 -> DVB-S2 LDPC Decoder_term2/1
  DVB-S2 BCH Decoder/2 -> ctrl/1

== system gm_soc_dvbs2_fpga/DVBS2/DVBS2 TxRx/DVB-S2 HDL Receiver/Demod Deinterleave and FECDecode/Symbol Demodulaor ==
  dataIn : Inport  OutDataTypeStr=fixdt(1, 18, 14)  PortDimensions=1  SampleTime=7.8125e-09
      settings: SignalType=complex
  validIn : Inport  Port=2  OutDataTypeStr=boolean  PortDimensions=1  SampleTime=7.8125e-09
  paramCapture : Inport  Port=3  OutDataTypeStr=boolean  PortDimensions=1  SampleTime=7.8125e-09
  modIdx : Inport  Port=4  OutDataTypeStr=fixdt(0, 2, 0)  PortDimensions=1  SampleTime=7.8125e-09
  codIdx : Inport  Port=5  OutDataTypeStr=fixdt(0, 4, 0)  PortDimensions=1  SampleTime=7.8125e-09
  FECFrame : Inport  Port=6  OutDataTypeStr=boolean  PortDimensions=1  SampleTime=7.8125e-09
  DVBS2 Symbol Demodulator : whdlmod/DVB-S2 Symbol Demodulator  ModulationSourceParams=Input port  ModulationScheme=QPSK  CodeRateAPSK=3/4  DecisionType=Approximate log-likelihood ratio  OutputType=Scalar  UnitAveragePower=off  EnbNoiseVar=off  SimulateUsing=Code generation
  DVBS2 Symbol Demodulator_term2 : Terminator
  Data Type Conversion : DataTypeConversion  OutDataTypeStr=fixdt(0,3,0)  SaturateOnIntegerOverflow=off  RndMeth=Floor
  Delay{1..4} (4 alike) : Delay  DelayLength=15
  softBitsOut : Outport  SampleTime=7.8125e-09
  validOut : Outport  Port=2  SampleTime=7.8125e-09
  paramCaptureOut : Outport  Port=3  SampleTime=7.8125e-09
  modIdxOut : Outport  Port=4  SampleTime=7.8125e-09
  codIdxOut : Outport  Port=5  SampleTime=7.8125e-09
  fecframeOut : Outport  Port=6  SampleTime=7.8125e-09
  wires:
  Delay3/1 -> fecframeOut/1
  FECFrame/1 -> Delay3/1
  paramCapture/1 -> Delay4/1
  Delay4/1 -> paramCaptureOut/1
  modIdx/1 -> Data Type Conversion/1, Delay1/1
  dataIn/1 -> DVBS2 Symbol Demodulator/1
  validIn/1 -> DVBS2 Symbol Demodulator/2
  Data Type Conversion/1 -> DVBS2 Symbol Demodulator/3
  DVBS2 Symbol Demodulator/2 -> validOut/1
  Delay1/1 -> modIdxOut/1
  codIdx/1 -> Delay2/1, DVBS2 Symbol Demodulator/4
  DVBS2 Symbol Demodulator/1 -> softBitsOut/1
  DVBS2 Symbol Demodulator/3 -> DVBS2 Symbol Demodulator_term2/1
  Delay2/1 -> codIdxOut/1
